simulink model "TEST_EdgeDetector_model"  (R2018b)
settings: Solver=VariableStepAuto  StartTime=0.0  StopTime=21  RelTol=1e-3
undefined symbols (not defined in the file): sigbuilder_block
libraries: dspswit3 x1
settings Model: Creator=Christopher  LastModifiedBy=Christopher

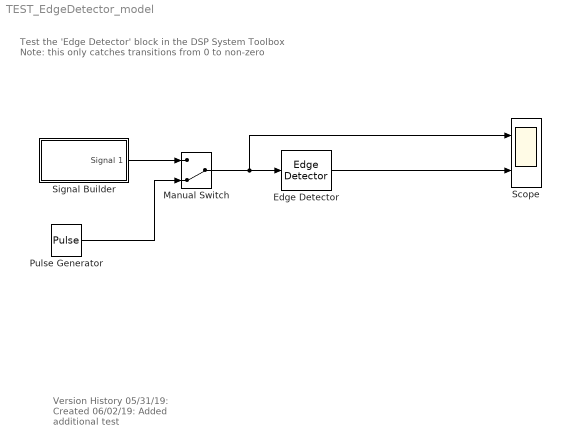
== system TEST_EdgeDetector_model ==
  note: Test the 'Edge Detector' block in the DSP System Toolbox
      |
      | Note: this only catches transitions from 0 to non-zero
  note: Version History
      | 05/31/19: Created
      | 06/02/19: Added additional test
  Edge Detector : dspswit3/Edge Detector  InputProcessing=Columns as channels (frame based)
      settings: SourceProductName=DSP System Toolbox  SourceProductBaseCode=DS
  Manual Switch : ManualSwitch  CurrentSetting=0
  Pulse Generator : DiscretePulseGenerator  PulseType=Time based  Period=10  PulseWidth=5
  Scope : Scope  NumInputPorts=2
  Signal Builder : Subsystem  Tag=STV Subsys  LoadFcn=sigbuilder_block('load',[-1440 900 1440 842.25 ]);  StartFcn=sigbuilder_block('start');  StopFcn=sigbuilder_block('stop');  ClipboardFcn=sigbuilder_block('clipboard');  mask(Sigbuilder block){tuvar=[0:10]}
      mask help: Simulink:masks:SigbuilderBlock_MD
      mask init:
      | if ~strcmp(get_param(bdroot(gcbh),'SimulationStatus'),'stopped') tuvar = sigbuilder_block('maskInit'); end
      settings: CopyFcn=sigbuilder_block('copy');  DeleteFcn=sigbuilder_block('delete');  ModelCloseFcn=sigbuilder_block('modelClose');  PreSaveFcn=sigbuilder_block('preSave');  PauseFcn=sigbuilder_block('pause');  ContinueFcn=sigbuilder_block('continue');  NameChangeFcn=sigbuilder_block('namechange');  OpenFcn=sigbuilder_block('open',[0 30 1440 812.25 ]);  CloseFcn=sigbuilder_block('close');
      mask Display: plot(0, 0, 100, 100,[2, 2, 32, 32, 2], [68, 8, 8, 68, 68],[32, 2], [38, 38], [32, 19, 2],[53, 60, 44], [32, 17, 17, 2],[16, 16, 31, 31]);txt = getActiveGroup(gcbh);text(2, 100, txt,'verticalAlignment', 'top');
  wires:
  Edge Detector/1 -> Scope/2
  Signal Builder/1(Signal 1) -> Manual Switch/1
  Pulse Generator/1 -> Manual Switch/2
  Manual Switch/1 -> Scope/1, Edge Detector/1

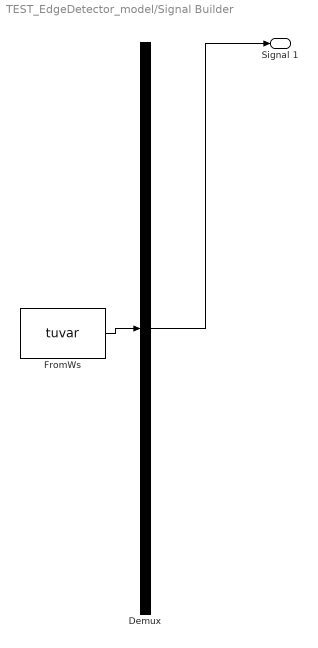
== system TEST_EdgeDetector_model/Signal Builder ==
  Demux : Demux  Tag=STV Demux  Outputs=1
  FromWs : FromWorkspace  Tag=STV FromWs  VariableName=tuvar  SampleTime=0
      SigBuilderData=|
      | common.afterFinalStr = 'Extrapolate'
      | common.sampleTime = 0
      | dataSet.timeRange = [0 10]
      | dataSet.name = 'Group 1'
      | sbobj.Groups.Name = 'Group 1'
      | sbobj.Groups.Signals.Name = 'Signal 1'
      | sbobj.Groups.Signals.XData = [0 1.82 1.82 2.54 2.54 3.99 3.99 5.72 6.96 7.55 8.64 9.38 10]
      | sbobj.Groups.Signals.YData = [0 0 1 1 0.5 0.5 0.498 0.8 -0.076 0.398 0 0 -0.5]
  Signal 1 : Outport  Tag=STV Outport
  wires:
  Demux/1 -> Signal 1/1
  FromWs/1 -> Demux/1
